simulink model "Disturbance_HIL"  (R2020a)
settings: Solver=ode4  StartTime=0.0  StopTime=100  FixedStep=0.01  RelTol=1e-3  EnableMultiTasking=on
values from neighbouring files (symbols this model uses):
  orbit0 = [r_ECI_0'; v_ECI_0']    [Disturbance_Initial.m]
  state0 = [wb; E_b_ECI'; quat_b_ECI]    [Disturbance_Initial.m]
  sun_ECI = [1; 0; 0]    [Disturbance_Initial.m]
  surfaceProperties = [Areas cps normals]    [Disturbance_Initial.m]
undefined symbols (not defined in the file or in its folder): Com2, IAU, none
libraries: xpcseriallib x6, aerolibtransform2 x1
settings Model: SimulationMode=external  Creator=sheab  LastModifiedBy=sheab
settings SolverCC: AutoInsertRateTranBlk=on
settings DataIOCC: SaveFormat=StructureWithTime  SaveOutput=off
settings OptimizationCC: BlockReduction=off  OptimizeBlockIOStorage=off
settings HardwareCC: ProdBitPerPointer=32  ProdBitPerSizeT=32  ProdBitPerPtrDiffT=32  ProdLargestAtomicFloat=None  ProdWordSize=32  ProdLongLongMode=on  ProdHWDeviceType=Generic->32-bit x86 compatible
settings RTWCC: Description=Simulink Real-Time  SystemTargetFile=slrt.tlc  TemplateMakefile=slrt_default_tmf  CodeExecutionProfiling=on  RTWCompilerOptimization=on
settings SimulinkRealTimeCC: SupportVariableSizeSignals=on  RL32LogTETModifier=off  xPCConcurrentTasks=on

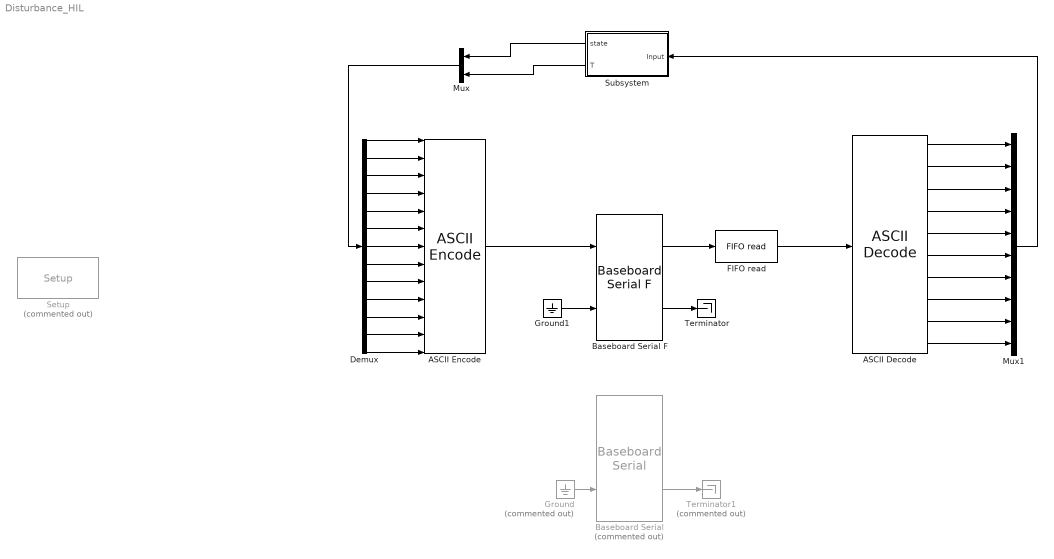
== system Disturbance_HIL ==
  "ASCII Decode " : xpcseriallib/ASCII Decode   format=%f %f %f %f %f %f %f %f %f %f\n  nvars=10  vartypes={}
      settings: SourceProductBaseCode=XP
  "ASCII Encode " : xpcseriallib/ASCII Encode   format=%.3f %.3f %.3f %.3f %.3f %.3f %.4f %.4f %.4f %.4f %.3e %.3e %.3e\n  nvars=13  maxlength=128  vartypes={ 'double' }
      settings: SourceProductBaseCode=XP
  Baseboard Serial : xpcseriallib/Mainboard/Baseboard Serial  Commented=on  group=Transmit Setup  port=1  irqnum=3  saddr1=0x2f8  saddr2=0x3e8  config=Com2/none  baud1=115200  parity1=None  ndata1=8  nstop1=1  fifomode1=64 deep  rlevel1=half full  automode1=on  xmtfifosize1=2048  xmtdatatype1=8 bit uint null terminated  rcvfifosize1=2048  rcvmaxread1=2048  rcvminread1=0  rcvusedelim1=on  rcvdelim1=10  rcvdatatype1=8 bit uint null terminated  rcvsampletime1=.05  baud2=115200  parity2=None  ndata2=8  nstop2=1  fifomode2=16 deep  rlevel2=half full  automode2=off  xmtfifosize2=1024  xmtdatatype2=8 bit uint null terminated  rcvfifosize2=1024  rcvmaxread2=1024  rcvminread2=1  rcvusedelim2=on  rcvdelim2=13  rcvdatatype2=count+16 bit uint  rcvsampletime2=.01
      settings: SourceProductBaseCode=XP
  Baseboard Serial F : xpcseriallib/Mainboard/Baseboard Serial F  group=FIFO Setup  port=1  irqnum=4  saddr1=0x3f8  saddr2=0x3e8  config=Com2/none  baud1=115200  parity1=None  ndata1=8  nstop1=1  fifomode1=16 deep  rlevel1=half full  automode1=off  xmtfifosize1=1024  xmtdatatype1=8 bit uint null terminated  rcvfifosize1=5120  baud2=115200  parity2=None  ndata2=8  nstop2=1  fifomode2=16 deep  rlevel2=half full  automode2=off  xmtfifosize2=1024  xmtdatatype2=8 bit uint null terminated  rcvfifosize2=1024
      settings: SourceProductBaseCode=XP
  Demux : Demux  Outputs=13
  "FIFO read " : xpcseriallib/FIFO read   maxsize=5028  minsize=1  usedelimiter=on  delimiter=10  outputtype=8 bit uint null terminated  enable=off  enableout=off  sampletime=0.01
      settings: SourceProductBaseCode=XP
  Ground : Ground  Commented=on
  Ground1 : Ground
  Mux : Mux  Inputs=2
  Mux1 : Mux  Inputs=10
  Setup : xpcseriallib/Mainboard/Baseboard Serial Internal  blocks/Setup  Commented=on  baud=115200  width=8  nstop=1  parity=None  fmode=16 deep  rlevel=half full  ctsmode=on  addr=0x2F8
      settings: SourceProductBaseCode=XP
  Subsystem : Subsystem
  Terminator : Terminator
  Terminator1 : Terminator  Commented=on
  wires:
  Ground/1 -> Baseboard Serial/2
  Baseboard Serial/2 -> Terminator1/1
  "ASCII Decode "/2 -> Mux1/2
  "ASCII Decode "/1 -> Mux1/1
  "ASCII Decode "/3 -> Mux1/3
  Ground1/1 -> Baseboard Serial F/2
  Baseboard Serial F/2 -> Terminator/1
  "ASCII Encode "/1 -> Baseboard Serial F/1
  "FIFO read "/1 -> "ASCII Decode "/1
  "ASCII Decode "/4 -> Mux1/4
  "ASCII Decode "/5 -> Mux1/5
  "ASCII Decode "/6 -> Mux1/6
  "ASCII Decode "/7 -> Mux1/7
  "ASCII Decode "/8 -> Mux1/8
  "ASCII Decode "/9 -> Mux1/9
  "ASCII Decode "/10 -> Mux1/10
  Baseboard Serial F/1 -> "FIFO read "/1
  Demux/1 -> "ASCII Encode "/1
  Demux/2 -> "ASCII Encode "/2
  Demux/3 -> "ASCII Encode "/3
  Demux/4 -> "ASCII Encode "/4
  Demux/5 -> "ASCII Encode "/5
  Demux/6 -> "ASCII Encode "/6
  Demux/7 -> "ASCII Encode "/7
  Demux/8 -> "ASCII Encode "/8
  Demux/9 -> "ASCII Encode "/9
  Demux/10 -> "ASCII Encode "/10
  Demux/11 -> "ASCII Encode "/11
  Demux/12 -> "ASCII Encode "/12
  Demux/13 -> "ASCII Encode "/13
  Subsystem/1(state) -> Mux/1
  Subsystem/2(T) -> Mux/2
  Mux/1 -> Demux/1
  Mux1/1 -> Subsystem/1(Input)

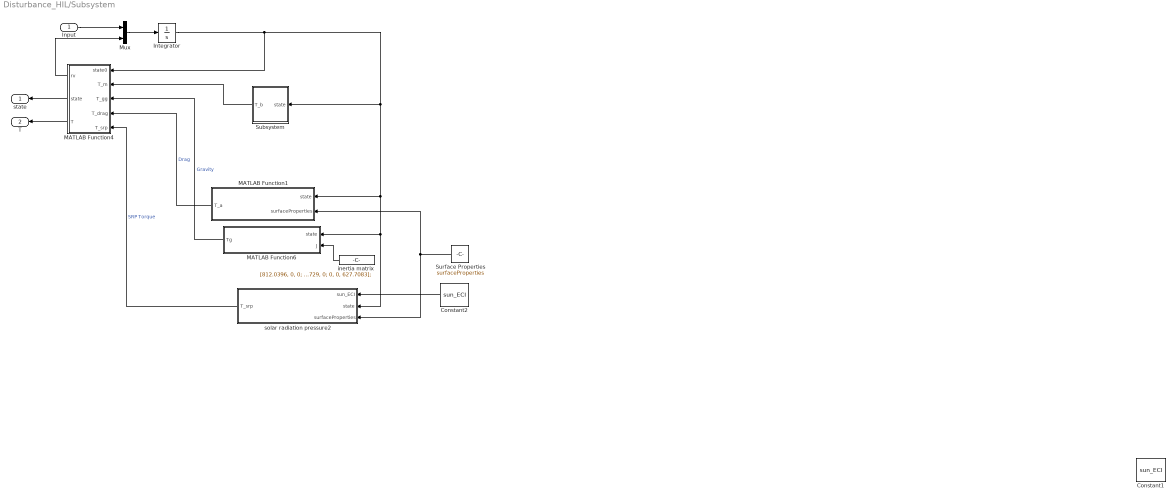
== system Disturbance_HIL/Subsystem ==
  Input : Inport
  Constant1 : Constant  Value=sun_ECI
  Constant2 : Constant  Value=sun_ECI
  Integrator : Integrator  InitialCondition=[state0; orbit0]  AbsoluteTolerance=10^(-8)  ZeroCross=off
  MATLAB Function1 : MATLAB Function  TreatAsAtomicUnit=on
  MATLAB Function4 : MATLAB Function  TreatAsAtomicUnit=on
  MATLAB Function6 : MATLAB Function  TreatAsAtomicUnit=on
  Mux : Mux  Inputs=2
  Subsystem : Subsystem
  Surface Properties : Constant  Value=surfaceProperties  VectorParams1D=off
  inertia matrix : Constant  Value=[812.0396, 0, 0; 0, 545.3729, 0; 0, 0, 627.7083];  VectorParams1D=off
  solar radiation pressure2 : MATLAB Function  TreatAsAtomicUnit=on
  state : Outport
  T : Outport  Port=2
  wires:
  Surface Properties/1 -> solar radiation pressure2/3(surfaceProperties), MATLAB Function1/2(surfaceProperties)
  inertia matrix/1 -> MATLAB Function6/2(J)
  Constant2/1 -> solar radiation pressure2/1(sun_ECI)
  MATLAB Function1/1(T_a) -> MATLAB Function4/4(T_drag)  "Drag"
  MATLAB Function6/1(Tg) -> MATLAB Function4/3(T_gg)  "Gravity"
  solar radiation pressure2/1(T_srp) -> MATLAB Function4/5(T_srp)  "SRP Torque"
  MATLAB Function4/3(T) -> T/1
  Mux/1 -> Integrator/1
  MATLAB Function4/1(rv) -> Mux/2
  Input/1 -> Mux/1
  MATLAB Function4/2(state) -> state/1
  Integrator/1 -> Subsystem/1(state), MATLAB Function1/1(state), solar radiation pressure2/2(state), MATLAB Function6/1(state), MATLAB Function4/1(state0)
  Subsystem/1(T_b) -> MATLAB Function4/2(T_m)

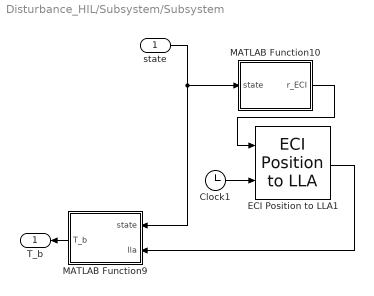
== system Disturbance_HIL/Subsystem/Subsystem ==
  state : Inport
  Clock1 : Clock
  ECI Position to LLA1 : aerolibtransform2/ECI Position to LLA  red=IAU-2000/2006  year=2020  month=March  day=20  hour=12  min=0  sec=0  deltaT=Sec  errorflag=Error  extraparamflag=off  eunits=Metric (MKS)  earthmodel=WGS84  flat=1/298.257223563  eqradius=6378137
      settings: AttributesFormatString=%<red>  SourceProductBaseCode=AE
  MATLAB Function10 : MATLAB Function  TreatAsAtomicUnit=on
  MATLAB Function9 : MATLAB Function  TreatAsAtomicUnit=on
  T_b : Outport
  wires:
  state/1 -> MATLAB Function10/1(state), MATLAB Function9/1(state)
  Clock1/1 -> ECI Position to LLA1/2
  ECI Position to LLA1/1 -> MATLAB Function9/2(lla)
  MATLAB Function10/1(r_ECI) -> ECI Position to LLA1/1
  MATLAB Function9/1(T_b) -> T_b/1

== matlab function Disturbance_HIL/Subsystem/MATLAB Function1 ==
  data: state input; T_a output; surfaceProperties input
function T_a  = atmosdrag(state, surfaceProperties)
q_b_ECI = [state(10); state(7); state(8); state(9)];
r_ECI = [state(11); state(12); state(13)];
v_ECI = [state(14); state(15); state(16)];

v_b = quat2rotm(q_b_ECI')*v_ECI;
Cd = 2.1;
Re = 6378.137;

rho_0 = 3.614e-14;
H = 88.667;
h_0 = 700;
nr = sqrt(r_ECI(1)^2 + r_ECI(2)^2 + r_ECI(3)^2);

density = rho_0*exp(-(nr - Re - h_0)/H);
T_a = zeros([3,1]);

nv = sqrt(v_ECI(1)^2 + v_ECI(2)^2 + v_ECI(3)^2);

for i = 1:length(surfaceProperties)
    A = surfaceProperties(i,1);
    cp = surfaceProperties(i,2:4);
    n = surfaceProperties(i,5:7);
    wet = n*v_b/sqrt(v_b(1)^2 + v_b(2)^2 + v_b(3)^2);
    if wet > 0
        A_wet = A*wet;
        v_b_hat = v_b/sqrt(v_b(1)^2 + v_b(2)^2 + v_b(3)^2);
        F_a = -1/2*density*(nv*1000)^2*Cd*A_wet*v_b_hat;
        T_a = T_a + cross(cp', F_a);
    end
end

== matlab function Disturbance_HIL/Subsystem/MATLAB Function4 ==
  data: rv output; state output; state0 input; T_m input; T_gg input; T_drag input; T_srp input; T output
function [rv, state, T] = attitude(state0, T_m, T_gg, T_drag, T_srp)
mu_earth = 398600;

% % initial state
w = [state0(1); state0(2); state0(3)];
% wx = [0, -w(3), w(2); w(3), 0, -w(1); -w(2), w(1), 0]; % omega cross
 epsilon = [state0(7); state0(8); state0(9)];
% epsilonx = [0, -epsilon(3), epsilon(2); epsilon(3), 0, -epsilon(1); -epsilon(2), epsilon(1), 0]; % epsilon cross
 eta = state0(10);
 phi = state0(4);
 theta = state0(5);
 psi = state0(6);

T = T_m + T_gg + T_drag + T_srp;

% derivatives
% wp = J^(-1)*(T - wx*J*w);
% epsilonp = 0.5*(eta*eye(3) + epsilonx)*w;
% etap = -0.5*epsilon'*w; % derivative of eta
% Ep = (1/cos(theta))*[cos(theta), sin(phi)*sin(theta), cos(phi)*sin(theta); ...
%     0, cos(phi)*cos(theta), -sin(phi)*cos(theta); ...
%     0, sin(phi), cos(phi)]*w; % E = [phi; theta; psi]

% initial state
rx = state0(11);
ry = state0(12);
rz = state0(13);
r = [rx; ry; rz];

rxp = state0(14);
ryp = state0(15);
rzp = state0(16);
rp = [rxp; ryp; rzp];

rxpp = -mu_earth*rx/norm(r)^3;
rypp = -mu_earth*ry/norm(r)^3;
rzpp = -mu_earth*rz/norm(r)^3;
rpp = [rxpp; rypp; rzpp];
% 
state = [w; E; epsilon; eta];

rv = [rp; rpp];

end

== matlab function Disturbance_HIL/Subsystem/MATLAB Function6 ==
  data: state input; Tg output; J input
function Tg = gravgrad(state, J)
muearth = 398600;

q_b_ECI = [state(10); state(7); state(7); state(9)];
r_ECI = [state(11); state(12); state(13)];

r_b = quat2rotm(q_b_ECI')*r_ECI;
r_b_x = [0, -r_b(3), r_b(2); r_b(3), 0, -r_b(1); -r_b(2), r_b(1), 0];

Tg = 3*muearth/sqrt(r_b(1)^2 + r_b(2)^2 + r_b(3)^2)^5*r_b_x*J*r_b;

end

== matlab function Disturbance_HIL/Subsystem/solar radiation pressure2 ==
  data: sun_ECI input; state input; surfaceProperties input; T_srp output
function T_srp = srp(sun_ECI, state, surfaceProperties)
% solar pressure (SRP)

p_sun = 4.5e-6; %N/m
q_b_ECI = [state(10); state(7); state(8); state(9)];

sun_b = quat2rotm(q_b_ECI')*sun_ECI;
T_srp = zeros([3,1]);
ns = sqrt(sun_b(1)^2 + sun_b(2)^2 + sun_b(3)^2);

%rho_sum = zeros([3,1]);
% Solar Radiation Pressure
for i = 1:length(surfaceProperties)
    A = surfaceProperties(i,1);
    cp = surfaceProperties(i,2:4);
    n = surfaceProperties(i,5:7);
    wet = n*sun_b/ns;
    if wet > 0
        A_wet = A*wet;
        F_srp = p_sun*A_wet*sun_b;
        T_srp = T_srp + cross(cp', F_srp);
        %rho_sum = rho_sum + rho';
    end
end

== matlab function Disturbance_HIL/Subsystem/Subsystem/MATLAB Function10 ==
  data: state input; r_ECI output
function r_ECI = postion(state)

r_ECI = [state(11); state(12); state(13)];

== matlab function Disturbance_HIL/Subsystem/Subsystem/MATLAB Function9 ==
  data: state input; T_b output; lla input
function T_b = wmm(state, lla)
m_b = 0.5*[0;0;-1];
m_bx = [0, -m_b(3), m_b(2); m_b(3), 0, -m_b(1); -m_b(2), m_b(1), 0];

%JD0 = 2458929.0;

%JD = JD0 + t/(24*3600);

a = 6371.2;
g_11 = -1450.9;
h_11 = 4652.5;
g_10 = -29404.8;

m_ECEF = a^3*[g_11; h_11; g_10];
m_ECEF = m_ECEF*1e-9*1000^3;

r_ECI = [state(11); state(12); state(13)]*1000;
r = norm(r_ECI);

long = lla(2);
angle = (-long*pi/180);
Cz = [cos(angle), -sin(angle), 0; sin(angle), cos(angle), 0; 0, 0, 1];

m_ECI = Cz*m_ECEF;

B_ECI = (3*m_ECI'*r_ECI*r_ECI - r^2*m_ECI)/r^5;

C_b_ECI = quat2rotm([state(10), state(7), state(8), state(9)]);

B_b = C_b_ECI*B_ECI;

T_b = m_bx*B_b;
